simulink model "sldemo_lct_start_term"  (Simulink 7.6)
settings: Solver=FixedStepDiscrete  StartTime=0.0  StopTime=20  FixedStep=0.01  RelTol=1e-3
Description:
  | Start and Terminate Actions
settings Model: Creator=The MathWorks Inc.  ExtModeAutoUpdateStatusClock=off
settings DataIOCC: SaveOutput=off  SaveTime=off  SignalLoggingName=sigsOut
settings OptimizationCC: InlineParams=on  InlineInvariantSignals=on  ZeroExternalMemoryAtStartup=off  ZeroInternalMemoryAtStartup=off  InitFltsAndDblsToZero=on  OptimizeModelRefInitCode=on  LifeSpan=1
settings DebuggingCC: SignalResolutionControl=TryResolveAllWithWarning  SolverPrmCheckMsg=none  MultiTaskDSMMsg=warning  MultiTaskCondExecSysMsg=none
settings HardwareCC: TargetUnknown=on
settings RTWCC: SystemTargetFile=ert.tlc  GenCodeOnly=on  TemplateMakefile=ert_default_tmf  Description=RTW Embedded Coder (no auto configuration)  GenerateReport=on  ProcessScript=ert_make_rtw_hook  IncludeHyperlinkInReport=on  LaunchReport=on  IncludeERTFirstTime=on
settings CodeAppCC: IgnoreCustomStorageClasses=off
settings ERTTargetCC: TargetFcnLib=ansi_tfl_tmw.mat  MultiwordLength=2048  GenerateSampleERTMain=on  InlinedParameterPlacement=NonHierarchical  ERTSrcFileBannerTemplate=example_banner.tlc  ERTHdrFileBannerTemplate=example_banner.tlc  ERTCustomFileTemplate=example_file_process.tlc  ConvertIfToSwitch=off

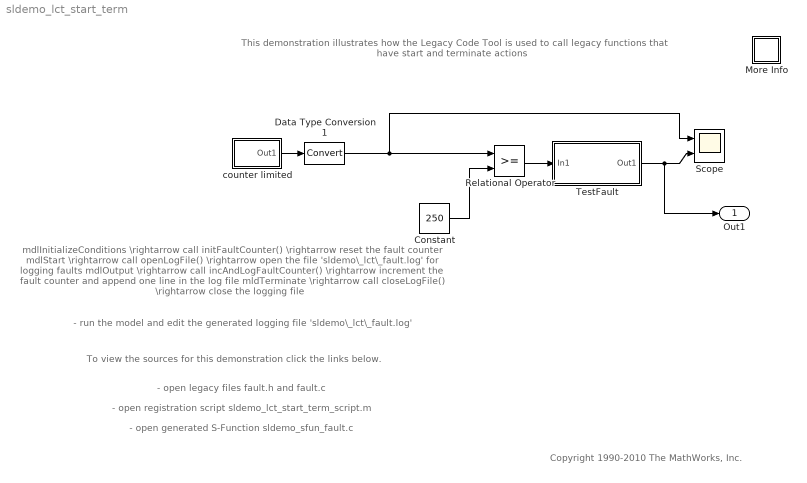
== system sldemo_lct_start_term ==
  note: mdlInitializeConditions \rightarrow call initFaultCounter() \rightarrow reset the fault counter
      | mdlStart  \rightarrow call openLogFile()   \rightarrow open the file 'sldemo\_lct\_fault.log' for logging faults
      | mdlOutput \rightarrow call incAndLogFaultCounter()  \rightarrow increment the fault counter and append one line in the log file
      | mldTerminate  \rightarrow call closeLogFile()  \rightarrow close the logging file
  note: Copyright 1990-2010 The MathWorks, Inc.
  note: This demonstration illustrates how the Legacy Code Tool is used to
      | call legacy functions that have start and terminate actions
  note: - open legacy files fault.h and fault.c
  note: To view the sources for this demonstration
      | click the links below.
  note: - open registration script sldemo_lct_start_term_script.m
  note: - open generated S-Function sldemo_sfun_fault.c
  note: - run the model and edit the generated logging file 'sldemo\_lct\_fault.log'
  Constant : Constant  Value=250
  Data Type Conversion1 : DataTypeConversion  RndMeth=Zero
  More Info : Subsystem
      settings: OpenFcn=showdemo('sldemo_lct_start_term_script')
      mask Display: disp('?')
  Relational Operator : RelationalOperator  OutDataTypeStr=boolean
  Scope : Scope  NumInputPorts=2
      settings: TimeRange=20  YMin=0~0  YMax=300~50
  TestFault : Subsystem
  counter limited : Subsystem  mask(CounterLimited){th=2^8-1}
      mask prompts: th "Threshold:"
  Out1 : Outport
  wires:
  TestFault/1(Out1) -> Out1/1, Scope/2
  counter limited/1(Out1) -> Data Type Conversion1/1
  Data Type Conversion1/1 -> Scope/1, Relational Operator/1
  Relational Operator/1 -> TestFault/1(In1)
  Constant/1 -> Relational Operator/2

== system sldemo_lct_start_term/More Info ==

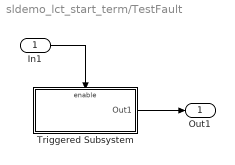
== system sldemo_lct_start_term/TestFault ==
  In1 : Inport
  Triggered Subsystem : Subsystem  TreatAsAtomicUnit=on
  Out1 : Outport
  wires:
  In1/1 -> Triggered Subsystem/Enable
  Triggered Subsystem/1(Out1) -> Out1/1

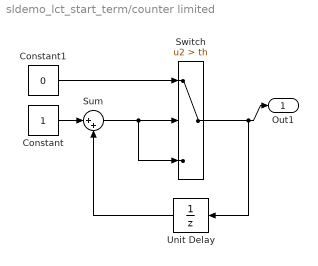
== system sldemo_lct_start_term/counter limited ==
  Constant : Constant
  Constant1 : Constant  Value=0
  Sum : Sum  Inputs=|++
  Switch : Switch  Criteria=u2 > Threshold  Threshold=th  ZeroCross=off
  Unit Delay : UnitDelay  X0=-1  SampleTime=-1
  Out1 : Outport
  wires:
  Constant/1 -> Sum/1
  Sum/1 -> Switch/2, Switch/3
  Unit Delay/1 -> Sum/2
  Constant1/1 -> Switch/1
  Switch/1 -> Unit Delay/1, Out1/1

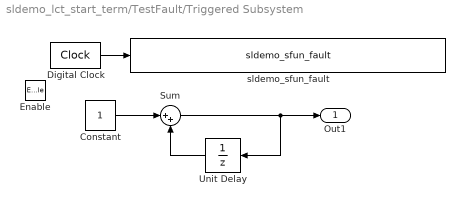
== system sldemo_lct_start_term/TestFault/Triggered Subsystem ==
  Enable : EnablePort
  Constant : Constant
  Digital Clock : DigitalClock  SampleTime=0.01
  Sum : Sum  Inputs=|++
  Unit Delay : UnitDelay  SampleTime=-1
  sldemo_sfun_fault : S-Function  FunctionName=sldemo_sfun_fault  EnableBusSupport=off  mask(Legacy Function){SFunctionSpec=incAndLogFaultCounter(void *work1, uint32 work2[1], double u1), ShowSpec=on}
      mask prompts: ShowSpec "Display function specification"
      mask help:
      | This block allows you to call the legacy functions specified by the following Legacy Code Tool definition:
      | def.SFunctionName = 'sldemo_sfun_fault';
      | def.InitializeConditionsFcnSpec = 'initFaultCounter(uint32 work2[1])';
      | def.OutputFcnSpec = 'incAndLogFaultCounter(void *work1, uint32 work2[1], double u1)';
      | def.StartFcnSpec = 'openLogFile(void **work1)';
      | def.TerminateFcnSpec = 'closeLogFile(void **work1)';
      | def.HeaderFiles = {'fault.h'};
      | def.SourceFiles = {'fault.c'};
      | def.IncPaths = {'sldemo_lct_src'};
      | def.SrcPaths = {'sldemo_lct_src'};
      | def.Options.useTlcWithAccel = false;
      mask Help: <p>This block was generated automatically by the Legacy Code Tool. For detailed help on this tool, call<a href="matlab:legacy_code('help')"> legacy_code('help')</a>.</p>
      mask CallbackString:
      | |if strcmp(get_param(gcbh, 'ShowSpec'), 'on')
      |   set_param(gcbh, 'MaskDisplay', sprintf('fprintf(''%s'');', get_param(gcbh, 'SFunctionSpec')));
      | else
      |   set_param(gcbh, 'MaskDisplay', sprintf('fprintf(''%s'');', get_param(gcbh, 'FunctionName')));
      | end
      mask Display: fprintf('incAndLogFaultCounter(void *work1, uint32 work2[1], double u1)');
  Out1 : Outport
  wires:
  Unit Delay/1 -> Sum/2
  Sum/1 -> Out1/1, Unit Delay/1
  Constant/1 -> Sum/1
  Digital Clock/1 -> sldemo_sfun_fault/1
